simulink model "Lotka_Vol"  (R2024b)
settings: Solver=VariableStepAuto  StartTime=0.0  StopTime=100.0  RelTol=1e-3
settings Model: Creator=Dario  LastModifiedBy=Dario
settings DataIOCC: ReturnWorkspaceOutputs=off  TimeSaveName=t

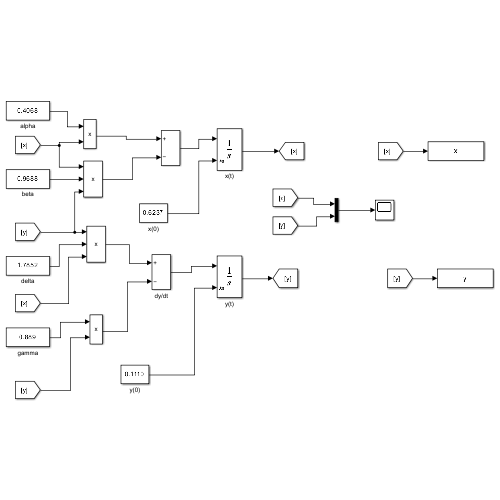
[thumbnail: Simulink's stored preview of the top-level diagram]
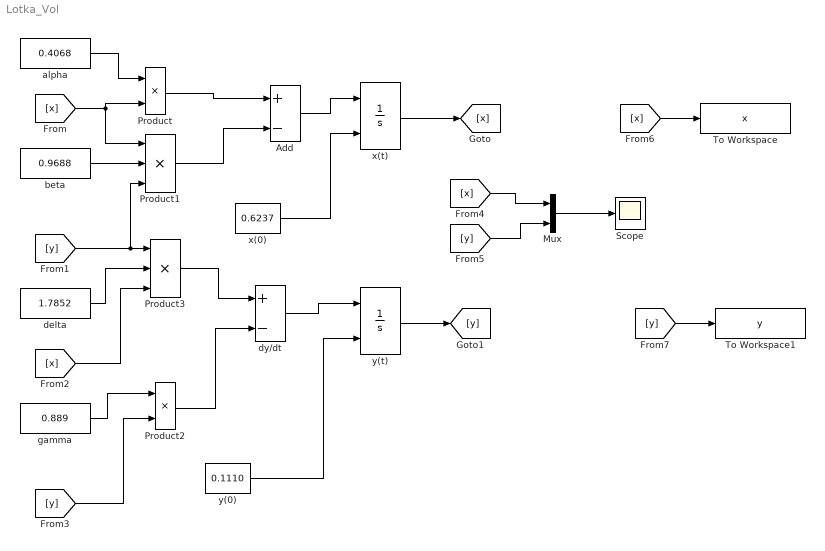
== system Lotka_Vol ==
  Add : Sum  Inputs=+-
  Mux : Mux  Inputs=2
  Product : Product
  Product1 : Product  Inputs=3
  Product2 : Product
  Product3 : Product  Inputs=3
  Scope : Scope
  To Workspace : ToWorkspace  VariableName=x  SampleTime=-1
  To Workspace1 : ToWorkspace  VariableName=y  SampleTime=-1
  alpha : Constant  Value=0.4068
  beta : Constant  Value=0.9688
  delta : Constant  Value=1.7852
  dy/dt : Sum  Inputs=+-
  gamma : Constant  Value=0.889
  x(0) : Constant  Value=0.6237
  x(t) : Integrator  InitialConditionSource=external
  y(0) : Constant  Value=0.1110
  y(t) : Integrator  InitialConditionSource=external
  wires:
  x(0)/1 -> x(t)/2
  dy/dt/1 -> y(t)/1
  y(0)/1 -> y(t)/2
  alpha/1 -> Product/1
  [y] -> Product2/2
  gamma/1 -> Product2/1
  [x] -> Product3/3
  delta/1 -> Product3/2
  [y] -> Product1/3, Product3/1
  beta/1 -> Product1/2
  [x] -> Product1/1, Product/2
  Product/1 -> Add/1
  Product1/1 -> Add/2
  Product3/1 -> dy/dt/1
  Product2/1 -> dy/dt/2
  y(t)/1 -> [y]
  x(t)/1 -> [x]
  [x] -> Mux/1
  [y] -> Mux/2
  Mux/1 -> Scope/1
  Add/1 -> x(t)/1
  [x] -> To Workspace/1
  [y] -> To Workspace1/1
